simulink model "smooth27"  (R2018b)
settings: Solver=VariableStepAuto  StartTime=0.0  StopTime=10.0  RelTol=1e-3
undefined symbols (not defined in the file or in its folder): gray
libraries: visionsources x1, visionstatistics x1
settings Model: Creator=Administrator  LastModifiedBy=Administrator
settings OptimizationCC: BlockReduction=off  ConditionallyExecuteInputs=off  DefaultParameterBehavior=Inlined
settings DebuggingCC: AlgebraicLoopMsg=error
settings HardwareCC: ProdBitPerPointer=32  ProdBitPerSizeT=32  ProdBitPerPtrDiffT=32  ProdLargestAtomicFloat=None  ProdIntDivRoundTo=Undefined  ProdEndianess=Unspecified  ProdWordSize=32  ProdHWDeviceType=ASIC/FPGA->ASIC/FPGA  TargetBitPerPointer=64  TargetBitPerSizeT=64  TargetBitPerPtrDiffT=64  TargetLongLongMode=on  TargetIntDivRoundTo=Zero  TargetEndianess=LittleEndian  TargetWordSize=64  TargetHWDeviceType=Custom Processor->MATLAB Host Computer  ProdEqTarget=off

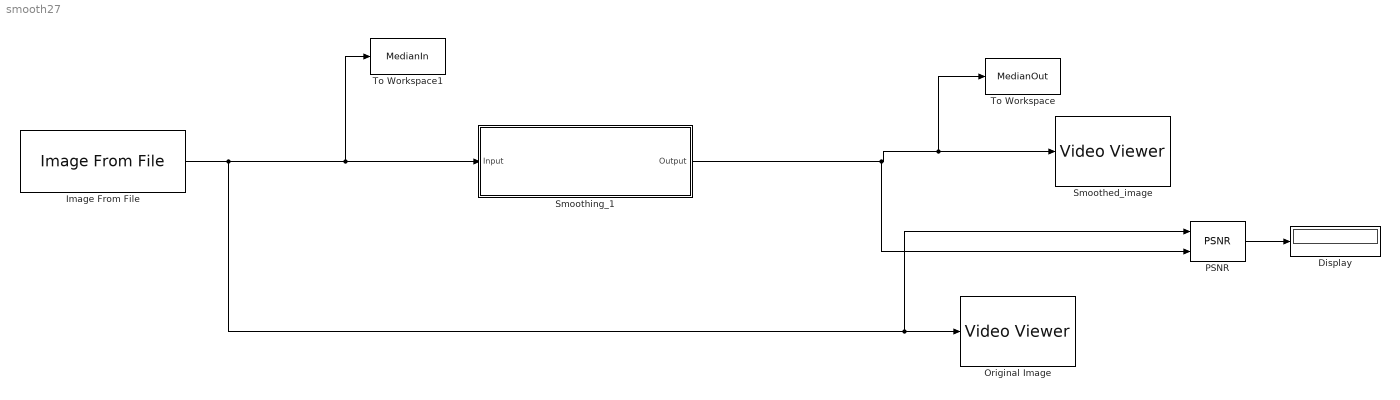
== system smooth27 ==
  Display : Display
  Image From File : visionsources/Image From File  Tag=vipblks_nd  FileName=C:\Users\Administrator\Desktop\chapter\101_4.tif  imagePorts=One multidimensional signal  Ts=0.1  ImageDataType=uint8  Signed=on  WordLength=16  sdImageDataType=uint(8)  FractionLengthMode=User-defined  FractionLength=15  OutPortLabels=R|G|B
      settings: SourceProductName=Computer Vision System Toolbox
  Original Image : VideoViewer  colormapValue=gray(256)  FigPos=[313 917 376 593]
  PSNR : visionstatistics/PSNR
      settings: SourceProductName=Computer Vision System Toolbox  SourceProductBaseCode=VP
  Smoothed_image : VideoViewer  colormapValue=gray(256)  FigPos=[708 876 361 543]
  Smoothing_1 : Subsystem  TreatAsAtomicUnit=on
  To Workspace : ToWorkspace  VariableName=MedianOut  SampleTime=-1
      settings: Save2DSignal=2-D array (concatenate along first dimension)
  To Workspace1 : ToWorkspace  VariableName=MedianIn  SampleTime=-1
      settings: Save2DSignal=2-D array (concatenate along first dimension)
  wires:
  Image From File/1 -> To Workspace1/1, Smoothing_1/1(Input), PSNR/1, Original Image/1
  Smoothing_1/1(Output) -> PSNR/2, To Workspace/1, Smoothed_image/1
  PSNR/1 -> Display/1

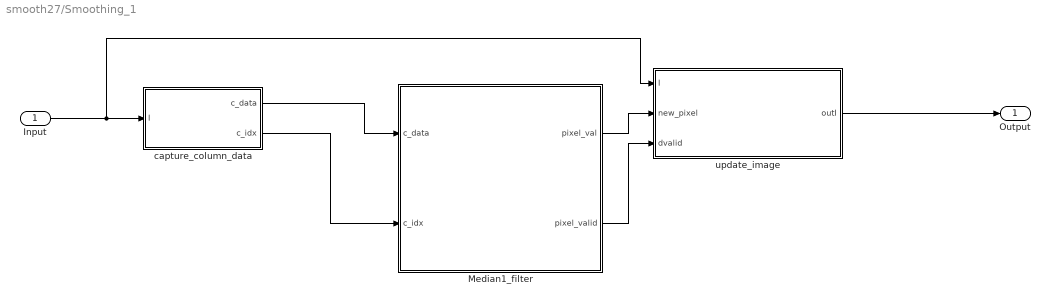
== system smooth27/Smoothing_1 ==
  Input : Inport
  Median1_filter : Subsystem  TreatAsAtomicUnit=on
  capture_column_data : MATLAB Function  TreatAsAtomicUnit=on
  update_image : MATLAB Function  TreatAsAtomicUnit=on
  Output : Outport
  wires:
  Input/1 -> update_image/1(I), capture_column_data/1(I)
  capture_column_data/1(c_data) -> Median1_filter/1(c_data)
  capture_column_data/2(c_idx) -> Median1_filter/2(c_idx)
  Median1_filter/2(pixel_valid) -> update_image/3(dvalid)
  Median1_filter/1(pixel_val) -> update_image/2(new_pixel)
  update_image/1(outI) -> Output/1

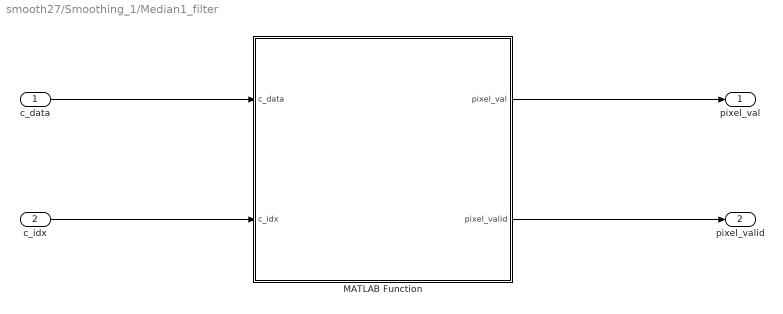
== system smooth27/Smoothing_1/Median1_filter ==
  c_data : Inport
  c_idx : Inport  Port=2
  MATLAB Function : MATLAB Function  TreatAsAtomicUnit=on
  pixel_val : Outport
  pixel_valid : Outport  Port=2
  wires:
  c_data/1 -> MATLAB Function/1(c_data)
  c_idx/1 -> MATLAB Function/2(c_idx)
  MATLAB Function/1(pixel_val) -> pixel_val/1
  MATLAB Function/2(pixel_valid) -> pixel_valid/1

== matlab function smooth27/Smoothing_1/Median1_filter/MATLAB Function ==
  data: c_data input; pixel_val output; c_idx input; pixel_valid output
%   Copyright 2011-2015 The MathWorks, Inc.

%I = imread('mlhdlc_img_pattern_noisy.tif');
% function J   = mlhdlc_median_filter_TB1(I)
% %I = imread('2_1.png');
% J = I;
% 
% smax = 9;
% [nrows, ncols] = size(I);
% ll = ceil(smax/2);
% ul = floor(smax/2);
% c_data = uint8(zeros(9,1));
% for ii=1:ncols-smax
%     for jj=1:nrows-smax
%         
%         c_idx = ii;                    
%         c_data = uint8(I(jj:jj+smax-1, ii));            
%         %coder.varsize('c_data');        
%         [pixel_val, pixel_valid] = mlhdlc_median_filter(c_data, c_idx);
%         
%         if pixel_valid
%             J(jj, ii) = pixel_val;
%         end
%     end
% end
% end

%#codegen
function [pixel_val, pixel_valid] = mlhdlc_median_filter(c_data, c_idx)

%   Copyright 2011-2015 The MathWorks, Inc.

smax = 9;
persistent window;
if isempty(window)
    window = zeros(smax, smax);
end

cp = ceil(smax/2); % center pixel;

w3 = -1:1;
w5 = -2:2;
w7 = -3:3;
w9 = -4:4;

r3 = cp + w3;      % 3x3 window
r5 = cp + w5;      % 5x5 window
r7 = cp + w7;      % 7x7 window
r9 = cp + w9;      % 9x9 window

d3x3 = window(r3, r3);
d5x5 = window(r5, r5);
d7x7 = window(r7, r7);
d9x9 = window(r9, r9);

center_pixel = window(cp, cp);


% use 1D filter for 3x3 region
outbuf = get_median_1d(d3x3(:)');
[min3, med3, max3] = getMinMaxMed_1d(outbuf);

% use 2D filter for 5x5 region
outbuf = get_median_2d(d5x5);
[min5, med5, max5] = getMinMaxMed_2d(outbuf);

% use 2D filter for 7x7 region
outbuf = get_median_2d(d7x7);
[min7, med7, max7] = getMinMaxMed_2d(outbuf);

% use 2D filter for 9x9 region
outbuf = get_median_2d(d9x9);
[min9, med9, max9] = getMinMaxMed_2d(outbuf);


pixel_val = get_new_pixel(min3, med3, max3, ...
    min5, med5, max5, ...
    min7, med7, max7, ...
    min9, med9, max9, ...
    center_pixel);


% we need to wait until 9 cycles for the buffer to fill up
% output is not valid every time we start from col1 for 9 cycles.
persistent datavalid
if isempty(datavalid)
    datavalid = false;
end
pixel_valid = datavalid;
datavalid = (c_idx >= smax);


% build the 9x9 buffer
window(:,2:smax) = window(:,1:smax-1);
window(:,1) = c_data;

end

%%%%%%%%%%%%%%%%%%%%%%%%%%%%%%%%%%%%%%%%%%%%%%%%%%%%%%%%%%%%%%%%%%%%%%%%%%%
function [min, med, max] = getMinMaxMed_1d(inbuf)

max = inbuf(1);
med = inbuf(ceil(numel(inbuf)/2));
min = inbuf(numel(inbuf));

end

%%%%%%%%%%%%%%%%%%%%%%%%%%%%%%%%%%%%%%%%%%%%%%%%%%%%%%%%%%%%%%%%%%%%%%%%%%%
function [min, med, max] = getMinMaxMed_2d(inbuf)

[nrows, ncols] = size(inbuf);
max = inbuf(1, 1);
med = inbuf(ceil(nrows/2), ceil(ncols/2));
min = inbuf(nrows, ncols);

end

%%%%%%%%%%%%%%%%%%%%%%%%%%%%%%%%%%%%%%%%%%%%%%%%%%%%%%%%%%%%%%%%%%%%%%%%%%%
function new_pixel  = get_new_pixel(...
    min3, med3, max3, ...
    min5, med5, max5, ...
    min7, med7, max7, ...
    min9, med9, max9, ...
    center_data)

if (med3 > min3 && med3 < max3)
    new_pixel = get_center_data(min3, med3, max3,center_data);
elseif (med5 > min5 && med5 < max5)
    new_pixel = get_center_data(min5, med5, max5,center_data);
elseif (med7 > min7 && med7 < max7)
    new_pixel = get_center_data(min7, med7, max7,center_data);
elseif (med9 > min9 && med9 < max9)
    new_pixel = get_center_data(min9, med9, max9,center_data);
else
    new_pixel = center_data;
end

end

%%%%%%%%%%%%%%%%%%%%%%%%%%%%%%%%%%%%%%%%%%%%%%%%%%%%%%%%%%%%%%%%%%%%%%%%%%%
function [new_data] = get_center_data(min,med,max,center_data)
if center_data <= min || center_data >= max
    new_data = med;
else
    new_data = center_data;
end
end

%%%%%%%%%%%%%%%%%%%%%%%%%%%%%%%%%%%%%%%%%%%%%%%%%%%%%%%%%%%%%%%%%%%%%%%%%%%
% perform median 1d computation
%%%%%%%%%%%%%%%%%%%%%%%%%%%%%%%%%%%%%%%%%%%%%%%%%%%%%%%%%%%%%%%%%%%%%%%%%%%
function outbuf = get_median_1d(inbuf)

numpixels = length(inbuf);

tbuf = inbuf;

for ii=coder.unroll(1:numpixels)
    if bitand(ii,uint32(1)) == 1  
        tbuf = compare_stage1(tbuf);
    else
        tbuf = compare_stage2(tbuf);
    end
end

outbuf = tbuf;

end

function outbuf = compare_stage1(inbuf)
numpixels = length(inbuf);
tbuf = compare_stage(inbuf(1:numpixels-1));
outbuf = [tbuf(:)' inbuf(numpixels)];
end

function outbuf = compare_stage2(inbuf)
numpixels = length(inbuf);
tbuf = compare_stage(inbuf(2:numpixels));
outbuf = [inbuf(1) tbuf(:)'];
end

function [outbuf] = compare_stage(inbuf)

step = 2;
numpixels = length(inbuf);

outbuf = inbuf;

for ii=coder.unroll(1:step:numpixels)
    t = compare_pixels([inbuf(ii), inbuf(ii+1)]);
    outbuf(ii) = t(1);
    outbuf(ii+1) = t(2);
end

end

function outbuf = compare_pixels(inbuf)
if (inbuf(1) > inbuf(2))
    outbuf = [inbuf(1), inbuf(2)];
else
    outbuf = [inbuf(2), inbuf(1)];
end
end


%%%%%%%%%%%%%%%%%%%%%%%%%%%%%%%%%%%%%%%%%%%%%%%%%%%%%%%%%%%%%%%%%%%%%%%%%%%
% perform median 2d computation
%%%%%%%%%%%%%%%%%%%%%%%%%%%%%%%%%%%%%%%%%%%%%%%%%%%%%%%%%%%%%%%%%%%%%%%%%%%
function outbuf = get_median_2d(inbuf)

outbuf = inbuf;
[nrows, ncols] = size(inbuf);
for ii=coder.unroll(1:ncols)
    colData = outbuf(:, ii)';
    colDataOut = get_median_1d(colData)';
    outbuf(:, ii) = colDataOut;
end
for ii=coder.unroll(1:nrows)
    rowData = outbuf(ii, :);
    rowDataOut = get_median_1d(rowData);
    outbuf(ii, :) = rowDataOut;
end

end

== matlab function smooth27/Smoothing_1/capture_column_data ==
  data: I input; c_data output; c_idx output
function [c_data, c_idx] = get_data(I)
% return a 1x9 column at a time from the Image

smax = 9;

[nrows, ncols] = size(I);

persistent col_idx;
persistent row_idx;

if isempty(row_idx)
    row_idx = uint32(1);
    col_idx = uint32(1);
end

c_idx = col_idx;

c_data = uint8(zeros(1,smax));

for ii=1:smax
    c_data(ii) = I(row_idx+ii-1, c_idx);
end


if (col_idx == ncols)
    col_idx = uint32(1);
    if (row_idx == nrows-smax+1)
        row_idx = uint32(1);
    else
        row_idx = row_idx+1;
    end
else
    col_idx = col_idx+1;
end

== matlab function smooth27/Smoothing_1/update_image ==
  data: I input; new_pixel input; dvalid input; outI output
function outI  = reconstruct_data(I, new_pixel, dvalid)

smax = 9;

% center pixel
cp = uint32(ceil(smax/2));

[nrows, ncols] = size(I);

persistent newI;
if isempty(newI)
    newI = I;
end

persistent col_idx;
persistent row_idx;

if isempty(row_idx)
    row_idx = cp;
    col_idx = cp;
end

outI = newI;

if dvalid == true
    newI(row_idx, col_idx) = new_pixel;
    
    if (col_idx == ncols-cp+1)
        col_idx = cp;
        if (row_idx == nrows-cp+1)
            row_idx = cp;
        else
            row_idx = row_idx+1;
        end
    else
        col_idx = col_idx+1;
    end
end
